simulink model "mpptproject_OandC_MPPT"  (R2025a)
settings: Solver=ode23t  StartTime=0.0  StopTime=100  RelTol=1e-3
libraries: fl_lib x6, nesl_utility x6, ee_lib x2
settings Model: Creator=jacks  LastModifiedBy=jacks

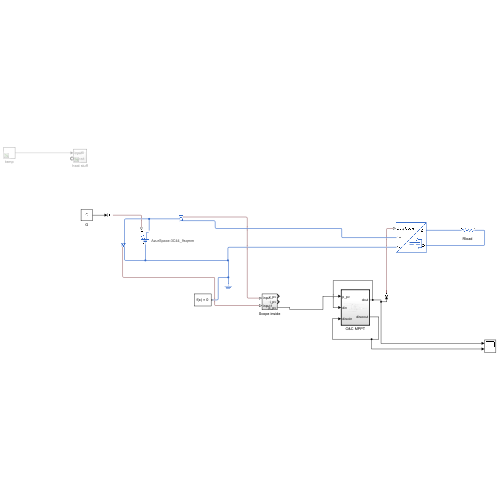
[thumbnail: Simulink's stored preview of the top-level diagram]
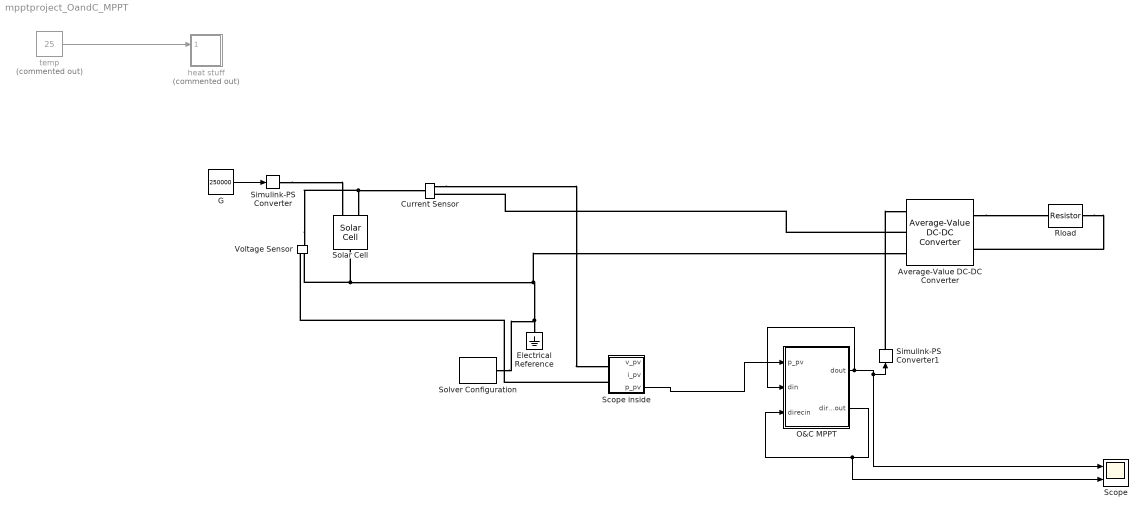
== system mpptproject_OandC_MPPT ==
  Average-Value DC-DC Converter : ee_lib/Semiconductors & Converters/Converters/Average-Value DC-DC Converter  implementation_option=ee.enum.converters.implementation.averageValue  converter_type=ee.enum.converters.dcdctype.boost  control_option=ee.enum.converters.controlinput.dutycycle  efficiency_option=ee.enum.converters.efficiency.constant  efficiency_fixed=100  i_vec=[0, 2, 5] A  efficiency_vec=[90, 95, 98]  Lf=100e-6 H  Rl=0 Ohm  Cf=100e-6 F  Rc=1e-6 Ohm  iL_specify=off  iL_priority=High  iL=0 A  iL_nominal_specify=off  iL_nominal_value=1  iL_nominal_unit=A  vc_specify=off  vc_priority=High  vc=0 V  vc_nominal_specify=off  vc_nominal_value=1  vc_nominal_unit=V
      settings: InternalSimscapePortConfiguration="{\"Bottom\":[],\"Left\":[{\"id\":\"DutyCycle\",\"label\":\"DutyCycle\",\"type\":\"input\"},{\"id\":\"p1\",\"label\":\"1+\",\"type\":\"foundation.electrical.electrical\"},{\"id\":\"n1\",\"label\":\"1-\",\"type\":\"foundation.electrical.electrical\"}],\"Right\":[{\"id\":\"p2\",\"label\":\"2+\",\"type\":\"foundation.electrical.electrical\"},{\"id\":\"n2\",\"label\":\"2-\",\"type\":\"foundation.electrical.electrical\"}],\"Top\":[]}"
  Current Sensor : fl_lib/Electrical/Electrical Sensors/Current Sensor
  Electrical Reference : fl_lib/Electrical/Electrical Elements/Electrical Reference
  G : Constant  Value=250000
  O&C MPPT : Subsystem  TreatAsAtomicUnit=on
  Rload : fl_lib/Electrical/Electrical Elements/Resistor  R=25 Ohm  i_specify=off  i_priority=None  i=0 A  i_nominal_specify=off  i_nominal_value=1  i_nominal_unit=A  v_specify=off  v_priority=None  v=0 V  v_nominal_specify=off  v_nominal_value=1  v_nominal_unit=V
  Scope : Scope  NumInputPorts=2
      settings: ActiveDisplayYMinimum=-2.3005794041550103  ActiveDisplayYMaximum=3.1566070667998347
  Scope inside : Subsystem
  Simulink-PS Converter : nesl_utility/Simulink-PS Converter  PhysicalDomain=network_engine_domain  SubClassName=ps_input  LeftPortType=input  RightPortType=output  PseudoPeriodic=off  Frequencies=[]  NoiseDistribution=none  NoiseParameters=[]  Unit=1  AffineConversion=off  FilteringAndDerivatives=provide  SimscapeFilterOrder=1  InputFilterTimeConstant=0.001  UdotUserProvided=0
  Simulink-PS Converter1 : nesl_utility/Simulink-PS Converter  PhysicalDomain=network_engine_domain  SubClassName=ps_input  LeftPortType=input  RightPortType=output  PseudoPeriodic=off  Frequencies=[]  NoiseDistribution=none  NoiseParameters=[]  Unit=1  AffineConversion=off  FilteringAndDerivatives=provide  SimscapeFilterOrder=1  InputFilterTimeConstant=0.001  UdotUserProvided=0
  Solar Cell : ee_lib/Sources/Solar Cell  PartSpecification="{\"CollectionId\":\"SimscapeElectrical\",\"CollectionVersion\":\"1.0.0\",\"DatasetId\":\"AzurSpace|3C44_9sqmm|simscape.electrical.solarCell\",\"DisplayName\":\"AzurSpace:3C44_9sqmm\"}"  prm=3  Isc=0.37 % Datasheet derived A  Voc=3.05 % Datasheet derived V  Is=1.91003784590348e-35 % Datasheet derived A  Is2=8.42205890783812e-38 % Datasheet derived A  Iph=0.370001258541474 % Datasheet derived A  Ir0=250000 % Datasheet derived W/m^2  ec=1.50364371134548 % Datasheet derived  N2=1.73316940278898 % Datasheet derived  Rs=0.306625056084457 % Datasheet derived Ohm  Rp=90147.3159723304 % Datasheet derived Ohm  N_series=1 % Datasheet derived  N_parallel=1 % Datasheet derived  TIPH1=0.000800010328673928 % Datasheet derived 1/K  EG=1.441 % Datasheet derived eV  TXIS1=104.115941100637 % Datasheet derived  TXIS2=5.57230100941371 % Datasheet derived  TRS1=0.775797800706674 % Datasheet derived  TRP1=0 % Parameter not set  Tmeas=25 % Datasheet derived degC  TFIXED=25 % Datasheet derived degC  thermal_mass=100 % Parameter not set J/K  initial_temperature=25 degC
      settings: AttributesFormatString=AzurSpace:3C44_9sqmm
  Solver Configuration : nesl_utility/Solver Configuration  PhysicalDomain=network_engine_domain  SubClassName=solver  LeftPortType=input  RightPortType=generic  Tones=[]  Harmonics=[]  SimulateNoise=off  Profile=off  UseLocalSampling=off  EnableSwitchedLinearOptims=on  FrequencyDomain=off  UseCCode=off  RelTol=0.001  AbsTol=0.001  MinStep=1e-09  ToWorkspace=off  RevertToSquareIcSolve=off  NumHomotopyIterations=100  PhasorMode=off  PhasorModeNumHarmonics=1  ConsistencySolver=NEWTON_XTOL_AFTER_FTOL  IndexReductionMethod=DerivativeReplacement  DoDC=off  ResidualTolerance=1e-09  ConsistencyTolSource=GLOBAL  ConsistencyAbsTol=0.001  ConsistencyRelTol=0.001  ConsistencyTolFactor=0.001  UseLocalSolver=off  LocalSolverChoice=NE_BACKWARD_EULER_ADVANCER  ResolveIndetEquations=on  FunctionEvalNumThread=1  LocalSolverSampleTime=0.001  DoFixedCost=off  MaxNonlinIter=3  MaxModeIter=2  ComputeImpulses=off  ImpulseIterations=2  LinearAlgebra=auto  LinearAlgebraNumThread=0  EquationFormulation=NE_TIME_EF  DelaysMemoryBudget=1024  AutomaticFiltering=on  FilteringTimeConstant=0.001  PartitionStorageMethod=AS_NEEDED  PartitionMemoryBudget=1024  PartitionMethod=ROBUST  MultibodyUseLocalSolver=off  MultibodyLocalSolverChoice=ODE1  MultibodyLocalSolverSampleTime=0.001
  Voltage Sensor : fl_lib/Electrical/Electrical Sensors/Voltage Sensor
  heat stuff : Subsystem  Commented=on
  temp : Constant  Commented=on  Value=25
  wires:
  G/1 -> Simulink-PS Converter/1
  temp/1 -> heat stuff/1(input0)
  Scope inside/3(p_pv) -> O&C MPPT/1(p_pv)
  O&C MPPT/1(dout) -> O&C MPPT/2(din), Scope/1, Simulink-PS Converter1/1
  O&C MPPT/2(direcout) -> Scope/2, O&C MPPT/3(direcin)
  connections:
  Simulink-PS Converter/RConn1 -- Solar Cell/LConn1
  Voltage Sensor/RConn2 -- Average-Value DC-DC Converter/LConn3 -- Solver Configuration/RConn1 -- Electrical Reference/LConn1 -- Solar Cell/RConn1
  Voltage Sensor/LConn1 -- Current Sensor/LConn1 -- Solar Cell/LConn2
  Current Sensor/RConn1 -- Scope inside/LConn1
  Scope inside/LConn2 -- Voltage Sensor/RConn1
  Simulink-PS Converter1/RConn1 -- Average-Value DC-DC Converter/LConn1
  Average-Value DC-DC Converter/RConn1 -- Rload/LConn1
  Average-Value DC-DC Converter/LConn2 -- Current Sensor/RConn2
  Rload/RConn1 -- Average-Value DC-DC Converter/RConn2

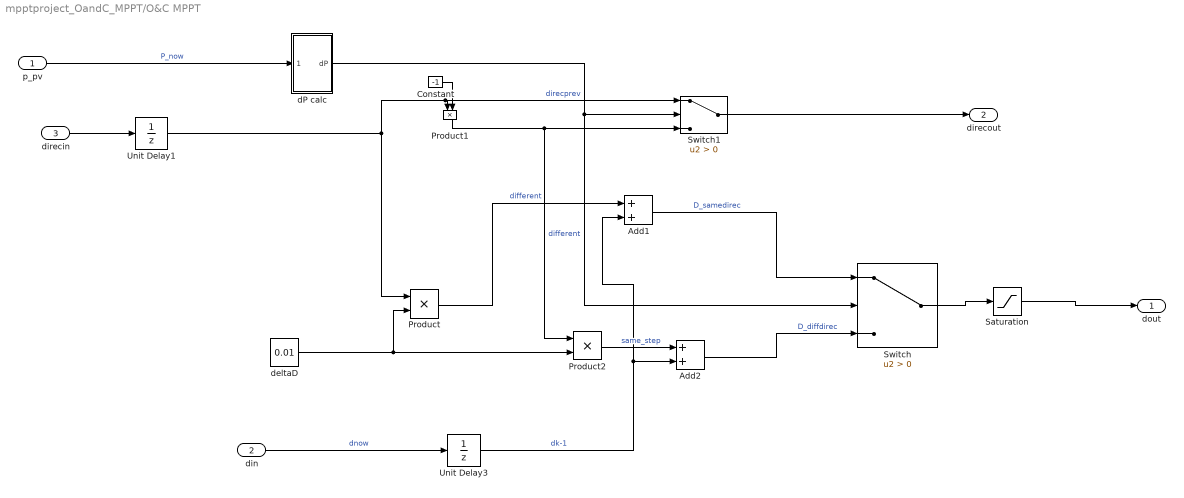
== system mpptproject_OandC_MPPT/O&C MPPT ==
  p_pv : Inport  SampleTime=0.001
  din : Inport  Port=2  SampleTime=0.001
  direcin : Inport  Port=3  SampleTime=0.001
  Add1 : Sum
  Add2 : Sum
  Constant : Constant  Value=-1
  Product : Product
  Product1 : Product
  Product2 : Product
  Saturation : Saturate  UpperLimit=0.95  LowerLimit=0.1
  Switch : Switch  Criteria=u2 > Threshold  ZeroCross=off  SaturateOnIntegerOverflow=off  InputSameDT=off
  Switch1 : Switch  Criteria=u2 > Threshold  ZeroCross=off  SaturateOnIntegerOverflow=off  InputSameDT=off
  Unit Delay1 : UnitDelay  InitialCondition=1  SampleTime=-1  HasFrameUpgradeWarning=on
  Unit Delay3 : UnitDelay  InitialCondition=0.3  SampleTime=-1  HasFrameUpgradeWarning=on
  dP calc : Subsystem
  deltaD : Constant  Value=0.01
  dout : Outport
  direcout : Outport  Port=2
  wires:
  din/1 -> Unit Delay3/1  "dnow"
  direcin/1 -> Unit Delay1/1
  Unit Delay1/1 -> Switch1/1, Product1/1, Product/1  "direcprev"
  Constant/1 -> Product1/2
  Product1/1 -> Product2/1, Switch1/3  "different"
  deltaD/1 -> Product2/2, Product/2
  Switch1/1 -> direcout/1
  Product/1 -> Add1/1  "different"
  Unit Delay3/1 -> Add1/2, Add2/2  "dk-1"
  Product2/1 -> Add2/1  "same_step"
  Add1/1 -> Switch/1  "D_samedirec"
  Add2/1 -> Switch/3  "D_diffdirec"
  dP calc/1(dP) -> Switch/2, Switch1/2
  p_pv/1 -> dP calc/1(P_now)  "P_now"
  Switch/1 -> Saturation/1
  Saturation/1 -> dout/1

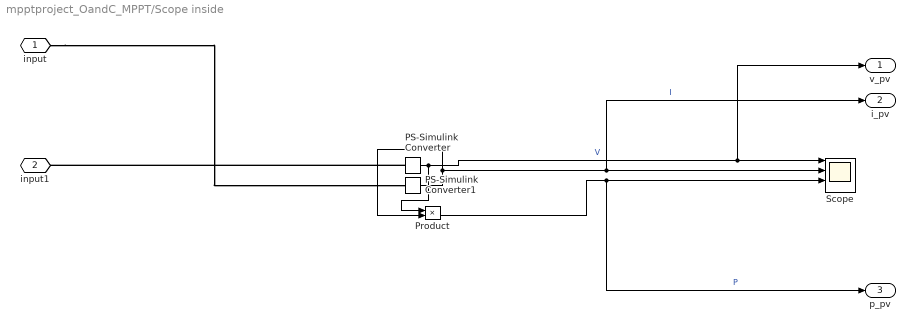
== system mpptproject_OandC_MPPT/Scope inside ==
  PS-Simulink Converter : nesl_utility/PS-Simulink Converter  PhysicalDomain=network_engine_domain  SubClassName=ps_output  LeftPortType=input  RightPortType=output  PseudoPeriodic=off  Frequencies=[]  VectorFormat=inherit  Unit=V  AffineConversion=off
  PS-Simulink Converter1 : nesl_utility/PS-Simulink Converter  PhysicalDomain=network_engine_domain  SubClassName=ps_output  LeftPortType=input  RightPortType=output  PseudoPeriodic=off  Frequencies=[]  VectorFormat=inherit  Unit=A  AffineConversion=off
  Product : Product
  Scope : Scope  NumInputPorts=4
      settings: ActiveDisplayYMinimum=-0.5022163740401524  ActiveDisplayYMaximum=4.1003859180090689
  input : PMIOPort  Side=Left
  input1 : PMIOPort  Port=2  Side=Left
  v_pv : Outport
  i_pv : Outport  Port=2
  p_pv : Outport  Port=3
  wires:
  PS-Simulink Converter/1 -> Product/1, v_pv/1, Scope/1  "V"
  PS-Simulink Converter1/1 -> Product/2, i_pv/1, Scope/2  "I"
  Product/1 -> p_pv/1, Scope/3  "P"
  connections:
  PS-Simulink Converter/LConn1 -- input1/RConn1
  input/RConn1 -- PS-Simulink Converter1/LConn1

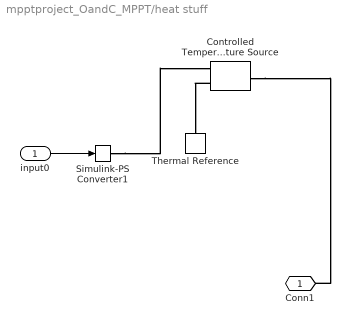
== system mpptproject_OandC_MPPT/heat stuff ==
  input0 : Inport
  Controlled Temperature Source : fl_lib/Thermal/Thermal Sources/Controlled Temperature Source
  Simulink-PS Converter1 : nesl_utility/Simulink-PS Converter  PhysicalDomain=network_engine_domain  SubClassName=ps_input  LeftPortType=input  RightPortType=output  PseudoPeriodic=off  Frequencies=[]  NoiseDistribution=none  NoiseParameters=[]  Unit=1  AffineConversion=off  FilteringAndDerivatives=provide  SimscapeFilterOrder=1  InputFilterTimeConstant=0.001  UdotUserProvided=0
  Thermal Reference : fl_lib/Thermal/Thermal Elements/Thermal Reference
  Conn1 : PMIOPort  Side=Left
  wires:
  input0/1 -> Simulink-PS Converter1/1
  connections:
  Controlled Temperature Source/RConn2 -- Thermal Reference/LConn1
  Simulink-PS Converter1/RConn1 -- Controlled Temperature Source/RConn1
  Controlled Temperature Source/LConn1 -- Conn1/RConn1

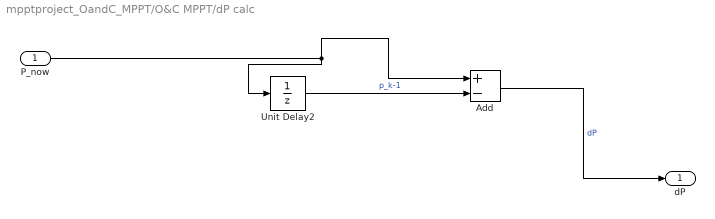
== system mpptproject_OandC_MPPT/O&C MPPT/dP calc ==
  P_now : Inport
  Add : Sum  Inputs=+-
  Unit Delay2 : UnitDelay  SampleTime=-1  HasFrameUpgradeWarning=on
  dP : Outport
  wires:
  Unit Delay2/1 -> Add/2  "p_k-1"
  P_now/1 -> Add/1, Unit Delay2/1
  Add/1 -> dP/1  "dP"
